simulink model "trab_sist_cont_modelo_planta_real"  (R2015a)
settings: Solver=ode45  StartTime=0.0  StopTime=10.0  RelTol=1e-3
settings Model: Creator=user  LastModifiedBy=user

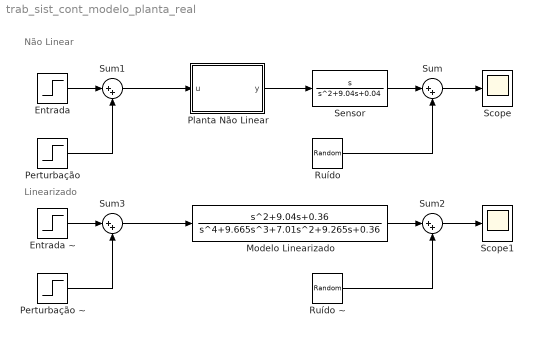
== system trab_sist_cont_modelo_planta_real ==
  note: Não Linear
  note: Linearizado
  Entrada : Step  SampleTime=0
  Entrada ~ : Step  SampleTime=0
  Modelo Linearizado : TransferFcn  Numerator=[1 9.04 0.36]  Denominator=[1 9.665 7.01 9.265 0.36]
  Perturbação : Step  SampleTime=0
  Perturbação ~ : Step  SampleTime=0
  Planta Não Linear : MATLAB Function  TreatAsAtomicUnit=on
  Ruído : RandomNumber  SampleTime=0.1
  Ruído ~ : RandomNumber  SampleTime=0.1
  Scope : Scope
  Scope1 : Scope
  Sensor : TransferFcn  Numerator=[1 0]  Denominator=[1 9.04 0.04]
  Sum{,1..3} (4 alike) : Sum  Inputs=|++
  wires:
  Entrada/1 -> Sum1/1
  Perturbação/1 -> Sum1/2
  Sum1/1 -> Planta Não Linear/1(u)
  Planta Não Linear/1(y) -> Sensor/1
  Sensor/1 -> Sum/1
  Sum/1 -> Scope/1
  Ruído/1 -> Sum/2
  Entrada ~/1 -> Sum3/1
  Perturbação ~/1 -> Sum3/2
  Sum3/1 -> Modelo Linearizado/1
  Modelo Linearizado/1 -> Sum2/1
  Sum2/1 -> Scope1/1
  Ruído ~/1 -> Sum2/2

== matlab function trab_sist_cont_modelo_planta_real/Planta Não Linear ==
  data: u input; y output
function y = fcn(u)
%#codegen

y = u;
